simulink model "Mohinhphanh1Acquy"  (R2024b)
settings: Solver=FixedStepAuto  StartTime=0  StopTime=2.08  FixedStep=0.0001  RelTol=1e-3  AbsTol=1e-3  EnableMultiTasking=on
undefined symbols (not defined in the file): a01, a02, a11, a12, b01, b02, b11, b12, h, J_bx, J_cl, K, km, m, r_bx, r_cl, rad, s, Trr
libraries: aerolibconvert2 x6, SignalEditorBlockLib x2
settings Model: Creator=Admin  LastModifiedBy=Legion
settings SolverCC: AutoScaleAbsTol=off  AlgebraicLoopSolver=TrustRegion  MaxZcPerStep=1
settings DataIOCC: LimitDataPoints=on  MaxDataPoints=10000
settings OptimizationCC: ReuseModelBlockBuffer=off  LifeSpan=inf
settings DebuggingCC: UnconnectedInputMsg=warning  UnconnectedOutputMsg=warning  UnconnectedLineMsg=warning  AllowSymbolicDim=off  SubsystemReferenceDiagnosticForUnitTest=warning  SFUnexpectedBacktrackingDiag=warning  SFNoUnconditionalDefaultTransitionDiag=warning  SFExecutionAtInitializationDiag=none  ArithmeticOperatorsInVariantConditions=warning
settings ModelReferenceCC: EnableRefExpFcnMdlSchedulingChecks=on
settings SFSimCC: SimUseLocalCustomCode=off  CustomCodeUndefinedFunction=UseInterfaceOnly
settings RTWCC: RTWUseLocalCustomCode=off  GPUComputeCapability=3.5  DLArmComputeVersion=19.05
settings CodeAppCC: StateflowObjectComments=on
settings GRTTargetCC: TargetLangStandard=C89/C90 (ANSI)
settings ConfigComp: CovMetricSettings=dw  CovSaveCumulativeToWorkspaceVar=on  CovSaveSingleToWorkspaceVar=on  CovExternalEMLEnable=off  CovSFcnEnable=off
settings SimscapeCC: SimscapeLogType=all  SimscapeLogSimulationStatistics=on  SimscapeLogDataHistory=10000

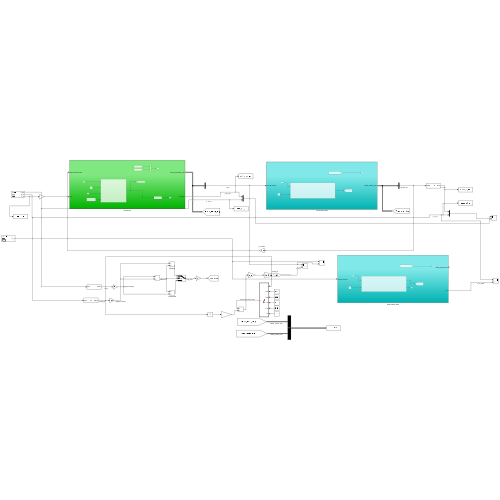
[thumbnail: Simulink's stored preview of the top-level diagram]
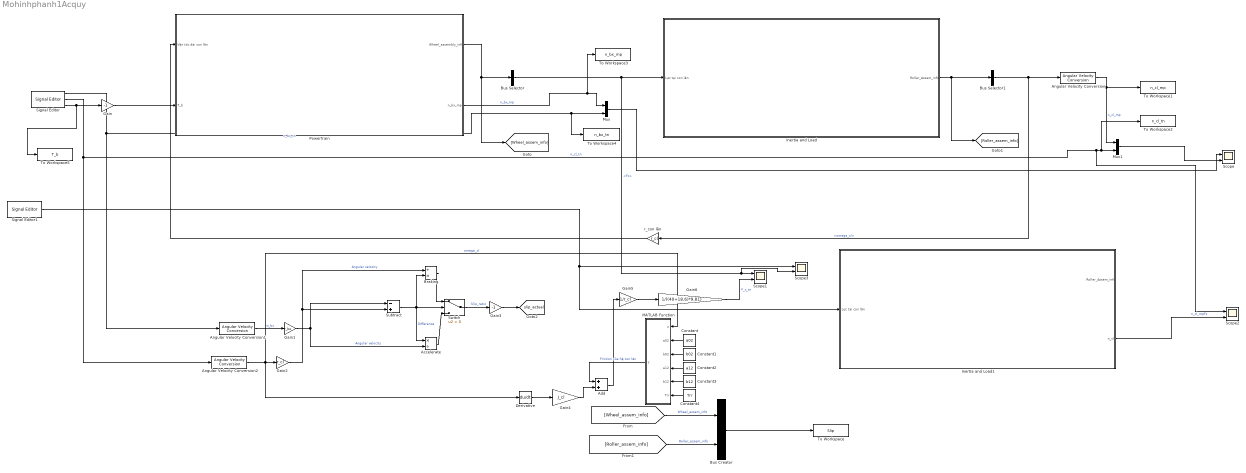
== system Mohinhphanh1Acquy ==
  " Inertia and Load" : Subsystem
  " Inertia and Load1" : Subsystem
  Accelerate : Product  Inputs=*/
  Add : Sum
  Angular Velocity Conversion : aerolibconvert2/Angular Velocity Conversion  IU=rad/s  OU=rpm
  Angular Velocity Conversion1 : aerolibconvert2/Angular Velocity Conversion  IU=rpm  OU=rad/s
  Angular Velocity Conversion2 : aerolibconvert2/Angular Velocity Conversion  IU=rpm  OU=rad/s
  Braking : Product  Inputs=/*
  Bus Creator : BusCreator  Inputs=2
  Bus Selector : BusSelector  OutputSignals=Wheel info.Fx
  Bus Selector1 : BusSelector  OutputSignals=omega_cl
  Constant : Constant  Value=a02
  Constant1 : Constant  Value=b02
  Constant2 : Constant  Value=a12
  Constant3 : Constant  Value=b12
  Constant4 : Constant  Value=Trr
  Derivative : Derivative
  Gain : Gain  Gain=-1
  Gain1 : Gain  Gain=r_bx
  Gain2 : Gain  Gain=r_cl
  Gain3 : Gain  Gain=-1
  Gain4 : Gain  Gain=J_cl
  Gain5 : Gain  Gain=1/r_cl
  Gain6 : Gain  Gain=1/((40+18.6)*9.81)
  MATLAB Function : MATLAB Function  TreatAsAtomicUnit=on
  Mux : Mux  Inputs=2
  Mux1 : Mux  Inputs=2
  Powertrain : Subsystem
  Scope{,1..3} (4 alike) : Scope  NumInputPorts=2
  Signal Editor : SignalEditorBlockLib/Signal Editor  FileName=DataPhanh1acquy.mat  ActiveScenario=Sheet1  ActiveSignal=n_bx  IsBus=off  OutputBusObjectStr=Bus: BusObject  SampleTime=0  ZeroCross=off  OutputAfterFinalValue=Setting to zero  Unit=inherit  PreserveSignalName=on  ApplySigPropsToAllScenarios=on  ApplySigPropsToAllSignals=off
  Signal Editor1 : SignalEditorBlockLib/Signal Editor  FileName=DataPhanh1acquy_Fx.mat  ActiveScenario=Sheet1  ActiveSignal=F_x  IsBus=off  OutputBusObjectStr=Bus: BusObject  SampleTime=0  Interpolate=off  ZeroCross=off  OutputAfterFinalValue=Setting to zero  Unit=inherit  PreserveSignalName=on  ApplySigPropsToAllScenarios=on  ApplySigPropsToAllSignals=off
  Subtract : Sum  Inputs=-+
  Switch : Switch  Criteria=u2 > Threshold  SaturateOnIntegerOverflow=off  InputSameDT=off
  To Workspace : ToWorkspace  VariableName=Slip  SaveFormat=Timeseries  SampleTime=-1
  To Workspace1 : ToWorkspace  VariableName=n_cl_mp  SaveFormat=Timeseries  SampleTime=-1
  To Workspace2 : ToWorkspace  VariableName=n_cl_tn  SaveFormat=Timeseries  SampleTime=-1
  To Workspace3 : ToWorkspace  VariableName=n_bx_mp  SaveFormat=Timeseries  SampleTime=-1
  To Workspace4 : ToWorkspace  VariableName=n_bx_tn  SaveFormat=Timeseries  SampleTime=-1
  To Workspace5 : ToWorkspace  VariableName=T_b  SaveFormat=Timeseries  SampleTime=-1
  r_con lăn : Gain  Gain=r_cl
  tag scope: slip_actual=global
  wires:
  Bus Selector/1 -> Scope3/2, Scope1/1, " Inertia and Load"/1(Lực tại con lăn)  "<Fx>"
  Powertrain/1(Wheel_assembly_info) -> Bus Selector/1, [Wheel_assem_info]
  " Inertia and Load"/1(Roller_Assem_info) -> [Roller_assem_info], Bus Selector1/1
  Bus Selector1/1 -> r_con lăn/1, Angular Velocity Conversion/1  "<omega_cl>"
  r_con lăn/1 -> Powertrain/1(Vận tốc dài con lăn)
  [Roller_assem_info] -> Bus Creator/2  "Roller_assem_info"
  [Wheel_assem_info] -> Bus Creator/1  "Wheel_assem_info"
  Bus Creator/1 -> To Workspace/1
  Powertrain/2(n_bx_mp) -> To Workspace3/1, Mux/1  "n_bx_mp"
  Angular Velocity Conversion/1 -> Mux1/1, To Workspace1/1  "n_cl_mp"
  Mux/1 -> Scope/1
  Signal Editor/3 -> To Workspace5/1, Gain/1
  Gain/1 -> Powertrain/2(T_b)
  Signal Editor/2 -> Angular Velocity Conversion2/1, Scope2/1, To Workspace2/1, Mux1/2  "n_cl_tn"
  Signal Editor/1 -> Angular Velocity Conversion1/1, To Workspace4/1, Mux/2  "n_bx_tn"
  Gain1/1 -> Accelerate/2, Subtract/1  "Angular velocity"
  Braking/1 -> Switch/1
  Subtract/1 -> Switch/2, Accelerate/1, Braking/2  "Difference"
  Accelerate/1 -> Switch/3
  Angular Velocity Conversion1/1 -> Gain1/1  "w_bx"
  Gain2/1 -> Subtract/2, Braking/1  "Angular velocity"
  Switch/1 -> Gain3/1  "Slip_ratio"
  Gain3/1 -> [slip_actual]
  Constant4/1 -> MATLAB Function/6(Trr)
  MATLAB Function/1(y) -> Add/1  "Friction của hệ con lăn"
  Angular Velocity Conversion2/1 -> Derivative/1, MATLAB Function/1(u), Gain2/1  "omega_cl"
  Constant3/1 -> MATLAB Function/5(b12)
  Constant1/1 -> MATLAB Function/3(b02)
  Constant/1 -> MATLAB Function/2(a02)
  Constant2/1 -> MATLAB Function/4(a12)
  Derivative/1 -> Gain4/1
  Gain4/1 -> Add/2
  Gain5/1 -> Gain6/1
  Add/1 -> Gain5/1
  Gain6/1 -> Scope1/2  "F_x_tn"
  Signal Editor1/1 -> " Inertia and Load1"/1(Lực tại con lăn), Scope3/1
  " Inertia and Load1"/2(n_cl) -> Scope2/2  "n_cl_mpFx"
  Mux1/1 -> Scope/2

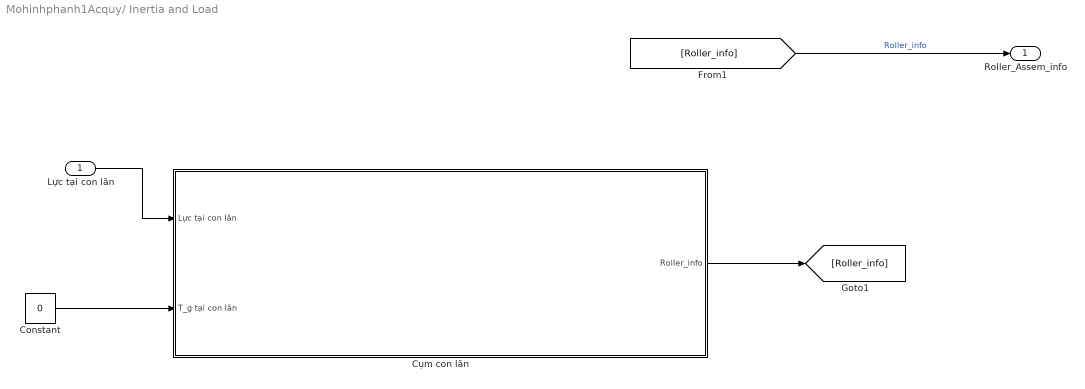
== system Mohinhphanh1Acquy/ Inertia and Load ==
  Lực tại con lăn : Inport
  Constant : Constant  Value=0
  Cụm con lăn : Subsystem
  Roller_Assem_info : Outport
  wires:
  Lực tại con lăn/1 -> Cụm con lăn/1(Lực tại con lăn)
  Cụm con lăn/1(Roller_info) -> [Roller_info]
  [Roller_info] -> Roller_Assem_info/1  "Roller_info"
  Constant/1 -> Cụm con lăn/2(T_g tại con lăn)

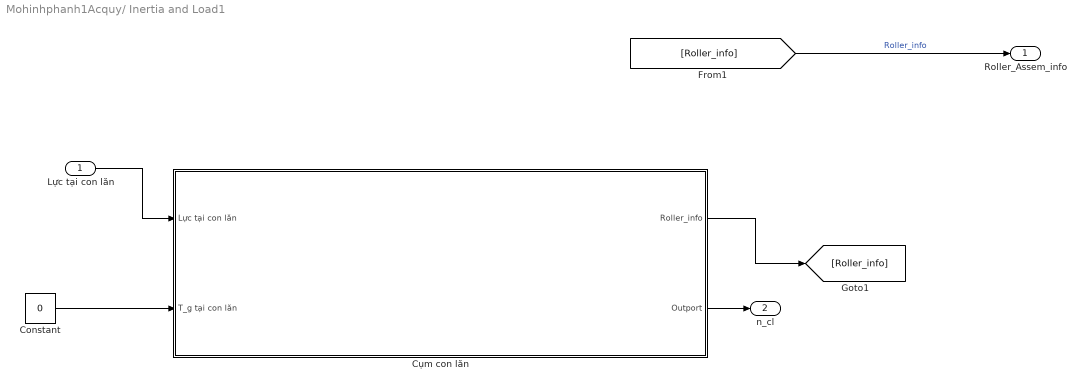
== system Mohinhphanh1Acquy/ Inertia and Load1 ==
  Lực tại con lăn : Inport
  Constant : Constant  Value=0
  Cụm con lăn : Subsystem
  Roller_Assem_info : Outport
  n_cl : Outport  Port=2
  wires:
  Lực tại con lăn/1 -> Cụm con lăn/1(Lực tại con lăn)
  Cụm con lăn/1(Roller_info) -> [Roller_info]
  [Roller_info] -> Roller_Assem_info/1  "Roller_info"
  Constant/1 -> Cụm con lăn/2(T_g tại con lăn)
  Cụm con lăn/2(Outport) -> n_cl/1

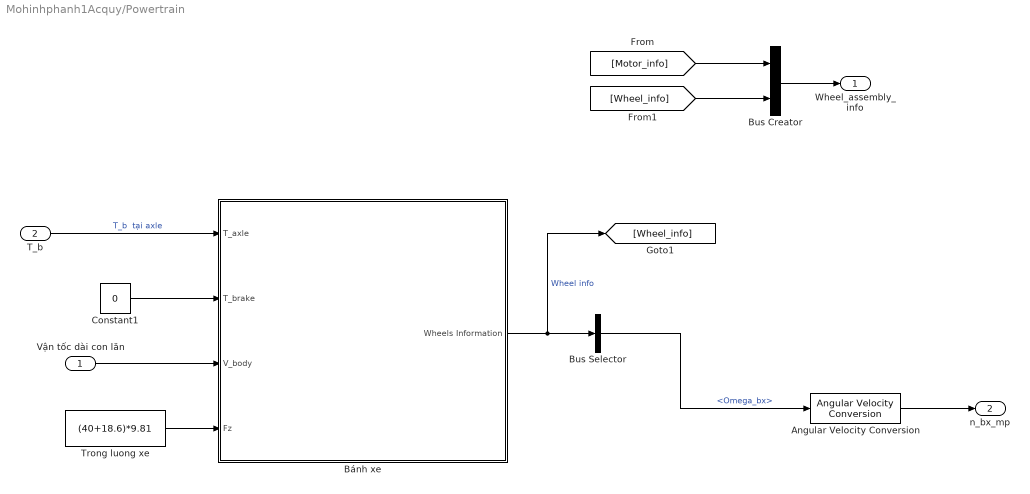
== system Mohinhphanh1Acquy/Powertrain ==
  Vận tốc dài con lăn : Inport
  T_b : Inport  Port=2
  Angular Velocity Conversion : aerolibconvert2/Angular Velocity Conversion  IU=rad/s  OU=rpm
  Bus Creator : BusCreator  Inputs=2
  Bus Selector : BusSelector  OutputSignals=Omega_bx
  Bánh xe : Subsystem
  Constant1 : Constant  Value=0
  Trong luong xe : Constant  Value=(40+18.6)*9.81
  Wheel_assembly_info : Outport
  n_bx_mp : Outport  Port=2
  wires:
  Bánh xe/1(Wheels Information) -> [Wheel_info], Bus Selector/1  "Wheel info"
  T_b/1 -> Bánh xe/1(T_axle)  "T_b  tại axle"
  Trong luong xe/1 -> Bánh xe/4(Fz)
  Constant1/1 -> Bánh xe/2(T_brake)
  Bus Selector/1 -> Angular Velocity Conversion/1  "<Omega_bx>"
  Vận tốc dài con lăn/1 -> Bánh xe/3(V_body)
  [Motor_info] -> Bus Creator/1
  [Wheel_info] -> Bus Creator/2
  Bus Creator/1 -> Wheel_assembly_info/1
  Angular Velocity Conversion/1 -> n_bx_mp/1

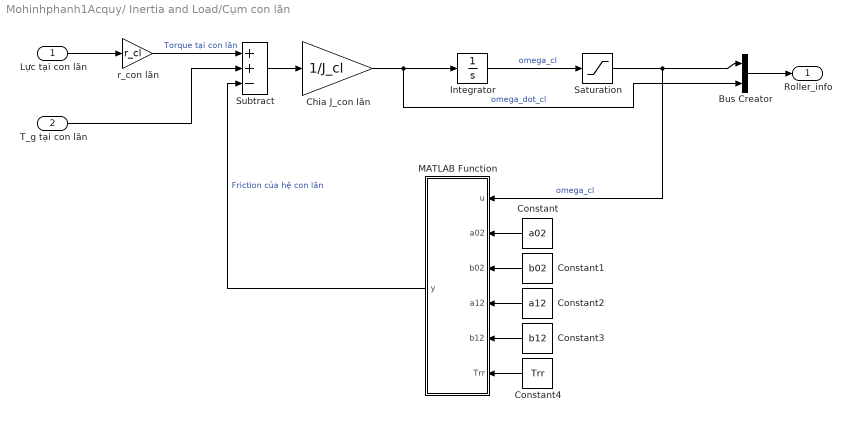
== system Mohinhphanh1Acquy/ Inertia and Load/Cụm con lăn ==
  Lực tại con lăn : Inport
  T_g tại con lăn : Inport  Port=2
  Bus Creator : BusCreator  Inputs=2
  Chia J_con lăn : Gain  Gain=1/J_cl
  Constant : Constant  Value=a02
  Constant1 : Constant  Value=b02
  Constant2 : Constant  Value=a12
  Constant3 : Constant  Value=b12
  Constant4 : Constant  Value=Trr
  Integrator : Integrator  InitialCondition=39.4364
  MATLAB Function : MATLAB Function  TreatAsAtomicUnit=on
  Saturation : Saturate  UpperLimit=inf  LowerLimit=0
  Subtract : Sum  Inputs=++-
  r_con lăn : Gain  Gain=r_cl
  Roller_info : Outport
  wires:
  Subtract/1 -> Chia J_con lăn/1
  r_con lăn/1 -> Subtract/1  "Torque tại con lăn"
  Saturation/1 -> Bus Creator/1, MATLAB Function/1(u)  "omega_cl"
  Integrator/1 -> Saturation/1  "omega_cl"
  Chia J_con lăn/1 -> Bus Creator/2, Integrator/1  "omega_dot_cl"
  MATLAB Function/1(y) -> Subtract/3  "Friction của hệ con lăn"
  T_g tại con lăn/1 -> Subtract/2
  Lực tại con lăn/1 -> r_con lăn/1
  Bus Creator/1 -> Roller_info/1
  Constant/1 -> MATLAB Function/2(a02)
  Constant1/1 -> MATLAB Function/3(b02)
  Constant2/1 -> MATLAB Function/4(a12)
  Constant3/1 -> MATLAB Function/5(b12)
  Constant4/1 -> MATLAB Function/6(Trr)

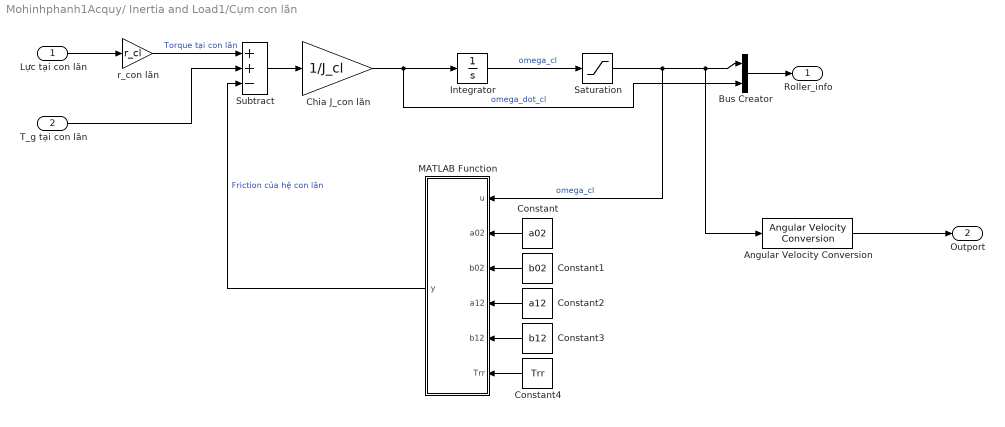
== system Mohinhphanh1Acquy/ Inertia and Load1/Cụm con lăn ==
  Lực tại con lăn : Inport
  T_g tại con lăn : Inport  Port=2
  Angular Velocity Conversion : aerolibconvert2/Angular Velocity Conversion  IU=rad/s  OU=rpm
  Bus Creator : BusCreator  Inputs=2
  Chia J_con lăn : Gain  Gain=1/J_cl
  Constant : Constant  Value=a02
  Constant1 : Constant  Value=b02
  Constant2 : Constant  Value=a12
  Constant3 : Constant  Value=b12
  Constant4 : Constant  Value=Trr
  Integrator : Integrator  InitialCondition=39.4364
  MATLAB Function : MATLAB Function  TreatAsAtomicUnit=on
  Saturation : Saturate  UpperLimit=inf  LowerLimit=0
  Subtract : Sum  Inputs=++-
  r_con lăn : Gain  Gain=r_cl
  Roller_info : Outport
  Outport : Outport  Port=2
  wires:
  Subtract/1 -> Chia J_con lăn/1
  r_con lăn/1 -> Subtract/1  "Torque tại con lăn"
  Saturation/1 -> Angular Velocity Conversion/1, Bus Creator/1, MATLAB Function/1(u)  "omega_cl"
  Integrator/1 -> Saturation/1  "omega_cl"
  Chia J_con lăn/1 -> Bus Creator/2, Integrator/1  "omega_dot_cl"
  MATLAB Function/1(y) -> Subtract/3  "Friction của hệ con lăn"
  T_g tại con lăn/1 -> Subtract/2
  Lực tại con lăn/1 -> r_con lăn/1
  Bus Creator/1 -> Roller_info/1
  Constant/1 -> MATLAB Function/2(a02)
  Constant1/1 -> MATLAB Function/3(b02)
  Constant2/1 -> MATLAB Function/4(a12)
  Constant3/1 -> MATLAB Function/5(b12)
  Constant4/1 -> MATLAB Function/6(Trr)
  Angular Velocity Conversion/1 -> Outport/1

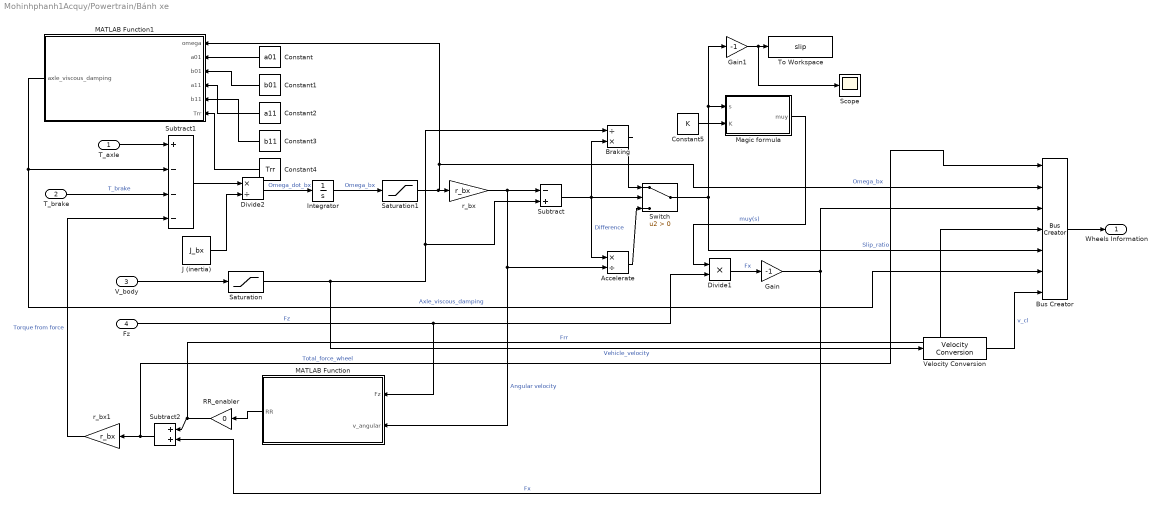
== system Mohinhphanh1Acquy/Powertrain/Bánh xe ==
  T_axle : Inport
  T_brake : Inport  Port=2
  V_body : Inport  Port=3
  Fz : Inport  Port=4
  Accelerate : Product  Inputs=*/
  Braking : Product  Inputs=/*
  Bus Creator : BusCreator  Inputs=7
  Constant : Constant  Value=a01
  Constant1 : Constant  Value=b01
  Constant2 : Constant  Value=a11
  Constant3 : Constant  Value=b11
  Constant4 : Constant  Value=Trr
  Constant5 : Constant  Value=K
  Divide1 : Product  Inputs=**
  Divide2 : Product  Inputs=*/
  Gain : Gain  Gain=-1
  Gain1 : Gain  Gain=-1
  Integrator : Integrator  InitialCondition=16.3518
  J (inertia) : Constant  Value=J_bx
  MATLAB Function : MATLAB Function  TreatAsAtomicUnit=on
  MATLAB Function1 : MATLAB Function  TreatAsAtomicUnit=on
  Magic formula : MATLAB Function  TreatAsAtomicUnit=on
  RR_enabler : Gain  Gain=0
  Saturation : Saturate  UpperLimit=inf  LowerLimit=0.00000000000000001
  Saturation1 : Saturate  UpperLimit=inf  LowerLimit=0.00000000000000001  ZeroCross=off
  Scope : Scope
  Subtract : Sum  Inputs=-+
  Subtract1 : Sum  Inputs=+---
  Subtract2 : Sum
  Switch : Switch  Criteria=u2 > Threshold  SaturateOnIntegerOverflow=off  InputSameDT=off
  To Workspace : ToWorkspace  VariableName=slip  SaveFormat=Timeseries  SampleTime=-1
  Velocity Conversion : aerolibconvert2/Velocity Conversion  IU=m/s  OU=km/h
  r_bx : Gain  Gain=r_bx
  r_bx1 : Gain  Gain=r_bx
  Wheels Information : Outport
  wires:
  Fz/1 -> Divide1/2, MATLAB Function/1(Fz)  "Fz"
  Subtract/1 -> Switch/2, Accelerate/1, Braking/2  "Difference"
  Saturation/1 -> Velocity Conversion/1, Braking/1, Subtract/2  "Vehicle_velocity"
  T_axle/1 -> Subtract1/1
  T_brake/1 -> Subtract1/3  "T_brake"
  Magic formula/1(muy) -> Divide1/1  "muy(s)"
  Accelerate/1 -> Switch/3
  Braking/1 -> Switch/1
  Switch/1 -> Bus Creator/5, Gain1/1, Magic formula/1(s)  "Slip_ratio"
  Subtract1/1 -> Divide2/1
  J (inertia)/1 -> Divide2/2
  Divide2/1 -> Integrator/1  "Omega_dot_bx"
  Divide1/1 -> Gain/1  "Fx"
  Gain/1 -> Bus Creator/3, Subtract2/2  "Fx"
  V_body/1 -> Saturation/1
  r_bx/1 -> Subtract/1, Accelerate/2, MATLAB Function/2(v_angular)  "Angular velocity"
  RR_enabler/1 -> Bus Creator/4, Subtract2/1  "Frr"
  MATLAB Function/1(RR) -> RR_enabler/1
  Subtract2/1 -> Bus Creator/1, r_bx1/1  "Total_force_wheel"
  r_bx1/1 -> Subtract1/4  "Torque from force"
  Saturation1/1 -> Bus Creator/2, MATLAB Function1/1(omega), r_bx/1  "Omega_bx"
  MATLAB Function1/1(axle_viscous_damping) -> Subtract1/2, Bus Creator/6  "Axle_viscous_damping"
  Integrator/1 -> Saturation1/1  "Omega_bx"
  Bus Creator/1 -> Wheels Information/1
  Velocity Conversion/1 -> Bus Creator/7  "v_cl"
  Constant/1 -> MATLAB Function1/2(a01)
  Constant1/1 -> MATLAB Function1/3(b01)
  Constant2/1 -> MATLAB Function1/4(a11)
  Constant3/1 -> MATLAB Function1/5(b11)
  Constant4/1 -> MATLAB Function1/6(Trr)
  Constant5/1 -> Magic formula/2(K)
  Gain1/1 -> Scope/1, To Workspace/1

== matlab function Mohinhphanh1Acquy/Powertrain/Bánh xe/MATLAB Function ==
  data: Fz input; RR output; v_angular input
function RR = rolling_resistance_function(Fz,v_angular)

RR = (0.015+7*10^(-6)*v_angular^2)*Fz;

== matlab function Mohinhphanh1Acquy/Powertrain/Bánh xe/Magic formula ==
  data: s input; muy output; K input
function muy = magicformula(s, K)
% Khai báo hằng số mặt đường
B = 12;
C = 2.3;
D = 0.82;
E = 1;
% Magic formula
muy = K * D * sin(C * atan(B * s - E * (B * s - atan(B * s))));

== matlab function Mohinhphanh1Acquy/Powertrain/Bánh xe/MATLAB Function1 ==
  data: omega input; axle_viscous_damping output; a01 input; b01 input; a11 input; b11 input; Trr input
function axle_viscous_damping = fcn(omega, a01, b01, a11, b11, Trr)
    axle_viscous_damping=0.0362*(a01*(omega)+b01)*15 + (a11*omega + b11) + Trr;

== matlab function Mohinhphanh1Acquy/ Inertia and Load/Cụm con lăn/MATLAB Function ==
  data: u input; y output; a02 input; b02 input; a12 input; b12 input; Trr input
function y = fcn(u,a02,b02,a12,b12,Trr)

y = 0.0362*(a02*u+b02)*2 + (a12*u+b12) + Trr;

== matlab function Mohinhphanh1Acquy/MATLAB Function ==
  data: u input; y output; a02 input; b02 input; a12 input; b12 input; Trr input
function y = fcn(u,a02,b02,a12,b12,Trr)

y = 0.0362*(a02*u+b02)*2 + (a12*u+b12) + Trr;

== matlab function Mohinhphanh1Acquy/ Inertia and Load1/Cụm con lăn/MATLAB Function ==
  data: u input; y output; a02 input; b02 input; a12 input; b12 input; Trr input
function y = fcn(u,a02,b02,a12,b12,Trr)

y = 0.0362*(a02*u+b02)*2 + (a12*u+b12) + Trr;
